simulink model "EPS_sim_test_v8a"  (R2023b)
settings: Solver=FixedStepAuto  StartTime=0.0  StopTime=tsimulation  FixedStep=delta_t  MaxStep=10  RelTol=1e-3
values from neighbouring files (symbols this model uses):
  ADCS =     [RWinfo.mat]
undefined symbols (not defined in the file or in its folder): Bat, Batt, EN, EPS, FIPEX, GPS, OBC, OCS, PL, UHF
libraries: simulink x4, cstextras x2
settings Model: Creator=Ricardo  LastModifiedBy=lricc
settings OptimizationCC: ReuseModelBlockBuffer=off
settings DebuggingCC: AlgebraicLoopMsg=none  UnconnectedInputMsg=warning  UnconnectedOutputMsg=warning  UnconnectedLineMsg=warning
settings ModelReferenceCC: EnableRefExpFcnMdlSchedulingChecks=on
settings SFSimCC: CustomCodeUndefinedFunction=UseInterfaceOnly
settings RTWCC: DLArmComputeVersion=19.05

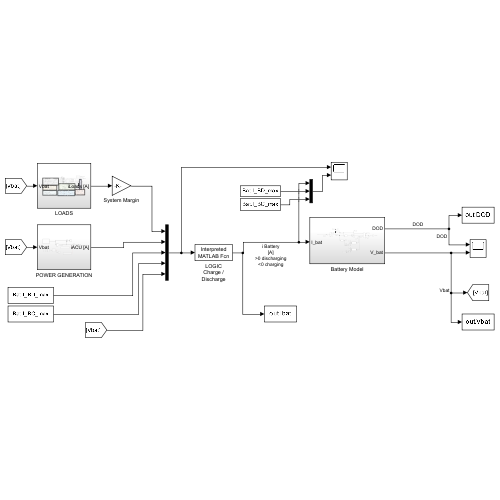
[thumbnail: Simulink's stored preview of the top-level diagram]
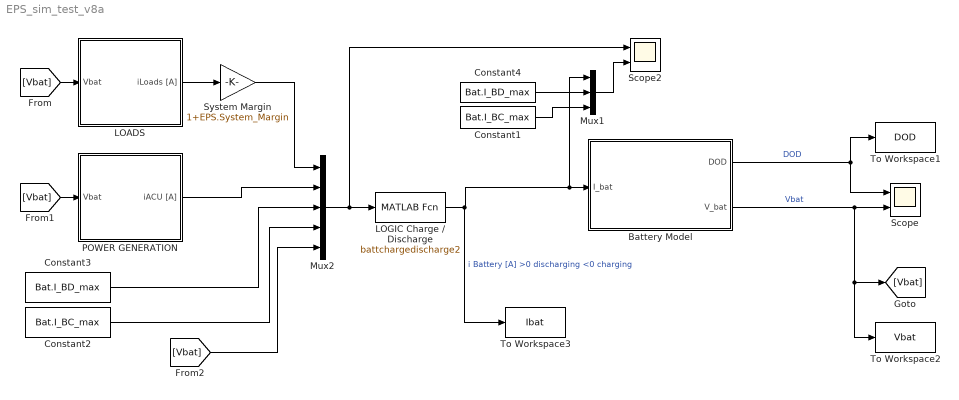
== system EPS_sim_test_v8a ==
  Battery Model : Subsystem
  Constant1 : Constant  Value=Bat.I_BC_max
  Constant2 : Constant  Value=Bat.I_BC_max
  Constant3 : Constant  Value=Bat.I_BD_max
  Constant4 : Constant  Value=Bat.I_BD_max
  LOADS : Subsystem
  LOGIC Charge / Discharge : MATLABFcn  MATLABFcn=battchargedischarge2
  Mux1 : Mux  Inputs=3
  Mux2 : Mux  Inputs=5
  POWER GENERATION : Subsystem
  Scope : Scope  NumInputPorts=2
  Scope2 : Scope  NumInputPorts=2
  System Margin : Gain  Gain=1+EPS.System_Margin
  To Workspace1 : ToWorkspace  VariableName=DOD  SaveFormat=Timeseries  SampleTime=-1
  To Workspace2 : ToWorkspace  VariableName=Vbat  SaveFormat=Timeseries  SampleTime=-1
  To Workspace3 : ToWorkspace  VariableName=Ibat  SaveFormat=Timeseries  SampleTime=-1
  wires:
  Battery Model/2(V_bat) -> [Vbat], To Workspace2/1, Scope/2  "Vbat"
  Battery Model/1(DOD) -> To Workspace1/1, Scope/1  "DOD"
  [Vbat] -> LOADS/1(Vbat)
  POWER GENERATION/1(iACU [A]) -> Mux2/2
  [Vbat] -> POWER GENERATION/1(Vbat)
  LOADS/1(iLoads [A]) -> System Margin/1
  Mux2/1 -> LOGIC Charge / Discharge/1, Scope2/1
  Constant3/1 -> Mux2/3
  Constant2/1 -> Mux2/4
  LOGIC Charge / Discharge/1 -> To Workspace3/1, Battery Model/1(I_bat), Mux1/1  "i Battery [A] >0 discharging <0 charging"
  [Vbat] -> Mux2/5
  Mux1/1 -> Scope2/2
  Constant4/1 -> Mux1/2
  Constant1/1 -> Mux1/3
  System Margin/1 -> Mux2/1

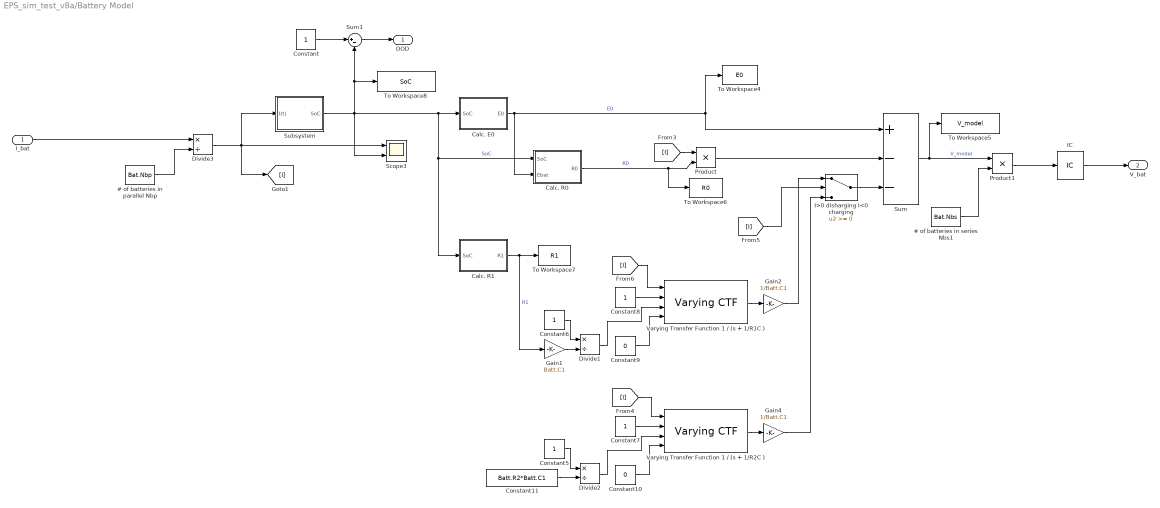
== system EPS_sim_test_v8a/Battery Model ==
  I_bat : Inport
  # of batteries in parallel Nbp : Constant  Value=Bat.Nbp
  # of batteries in series Nbs1 : Constant  Value=Bat.Nbs
  Calc. E0 : MATLAB Function  TreatAsAtomicUnit=on
  Calc. R0 : MATLAB Function  TreatAsAtomicUnit=on
  Calc. R1 : MATLAB Function  TreatAsAtomicUnit=on
  Constant{,5..8} (5 alike) : Constant
  Constant10 : Constant  Value=0
  Constant11 : Constant  Value=Batt.R2*Batt.C1
  Constant9 : Constant  Value=0
  Divide1 : Product  Inputs=*/
  Divide2 : Product  Inputs=*/
  Divide3 : Product  Inputs=*/
  Gain1 : Gain  Gain=Batt.C1
  Gain2 : Gain  Gain=1/Batt.C1
  Gain4 : Gain  Gain=1/Batt.C1
  I>0 disharging I<0 charging : Switch  SaturateOnIntegerOverflow=off  InputSameDT=off
  IC : InitialCondition  Value=4
  Product : Product
  Product1 : Product
  Scope3 : Scope  NumInputPorts=2
  Subsystem : Subsystem
  Sum : Sum  Inputs=+--
  Sum1 : Sum  Inputs=|+-
  To Workspace4 : ToWorkspace  VariableName=E0  SaveFormat=Timeseries  SampleTime=-1
  To Workspace5 : ToWorkspace  VariableName=V_model  SaveFormat=Timeseries  SampleTime=-1
  To Workspace6 : ToWorkspace  VariableName=R0  SaveFormat=Timeseries  SampleTime=-1
  To Workspace7 : ToWorkspace  VariableName=R1  SaveFormat=Timeseries  SampleTime=-1
  To Workspace8 : ToWorkspace  VariableName=SoC  SaveFormat=Timeseries  SampleTime=-1
  Varying Transfer Function 1 / (s + 1/R1C ) : cstextras/Varying CTF  N=1
  Varying Transfer Function 1 / (s + 1/R2C ) : cstextras/Varying CTF  N=1
  DOD : Outport
  V_bat : Outport  Port=2
  wires:
  Varying Transfer Function 1 / (s + 1/R2C )/1 -> Gain4/1
  Constant11/1 -> Divide2/2
  [I] -> Product/1
  Calc. E0/1(E0) -> To Workspace4/1, Sum/1, Calc. R0/2(Ebat)  "E0"
  # of batteries in parallel Nbp/1 -> Divide3/2
  [I] -> I>0 disharging I<0 charging/2
  Divide3/1 -> [I], Subsystem/1(I(t)), Scope3/1
  Calc. R1/1(R1) -> To Workspace7/1, Gain1/1  "R1"
  Calc. R0/1(R0) -> To Workspace6/1, Product/2  "R0"
  Subsystem/1(SoC) -> Sum1/2, To Workspace8/1, Calc. R1/1(SoC), Calc. R0/1(SoC), Calc. E0/1(SoC), Scope3/2  "SoC"
  Product/1 -> Sum/2
  [I] -> Varying Transfer Function 1 / (s + 1/R2C )/1
  Gain4/1 -> I>0 disharging I<0 charging/3
  Sum/1 -> To Workspace5/1, Product1/1  "V_model"
  Constant10/1 -> Varying Transfer Function 1 / (s + 1/R2C )/4
  Gain2/1 -> I>0 disharging I<0 charging/1
  Constant5/1 -> Divide2/1
  Constant8/1 -> Varying Transfer Function 1 / (s + 1/R1C )/2
  Varying Transfer Function 1 / (s + 1/R1C )/1 -> Gain2/1
  [I] -> Varying Transfer Function 1 / (s + 1/R1C )/1
  Constant6/1 -> Divide1/1
  Constant7/1 -> Varying Transfer Function 1 / (s + 1/R2C )/2
  Divide1/1 -> Varying Transfer Function 1 / (s + 1/R1C )/3
  Constant9/1 -> Varying Transfer Function 1 / (s + 1/R1C )/4
  I>0 disharging I<0 charging/1 -> Sum/3
  Product1/1 -> IC/1
  Gain1/1 -> Divide1/2
  Divide2/1 -> Varying Transfer Function 1 / (s + 1/R2C )/3
  # of batteries in series Nbs1/1 -> Product1/2
  I_bat/1 -> Divide3/1
  Constant/1 -> Sum1/1
  Sum1/1 -> DOD/1
  IC/1 -> V_bat/1

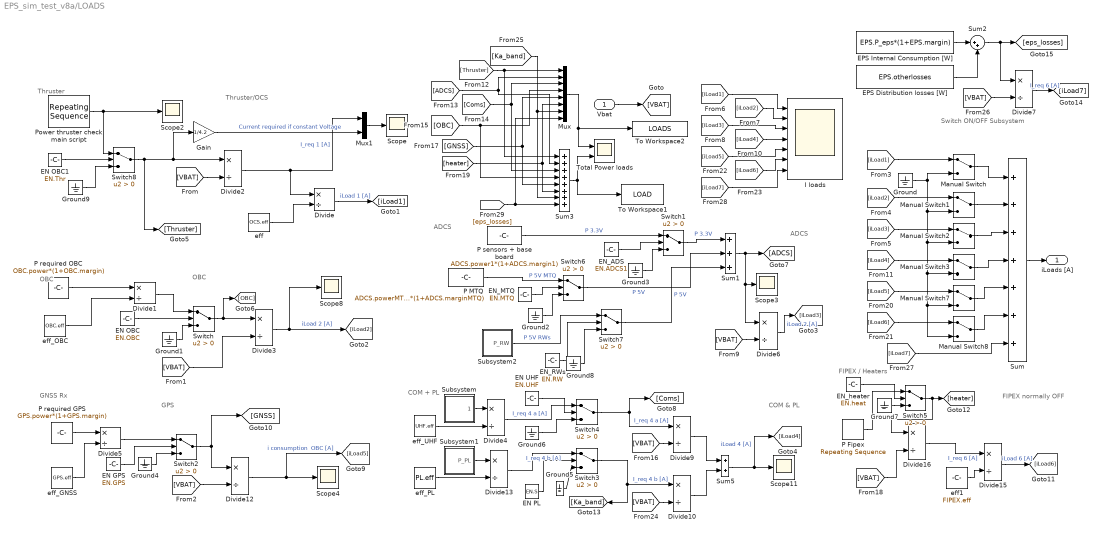
== system EPS_sim_test_v8a/LOADS ==
  note: Switch
      | ON/OFF
      | Subsystem
  note: FIPEX / Heaters
  note: COM + PL
  note: ADCS
  note: OBC
  note: Thruster
  note: Thruster/OCS
  note: OBC
  note: ADCS
  note: COM & PL
  note: GPS
  note: GNSS Rx
  note: FIPEX
      | normally
      | OFF
  Vbat : Inport
  Divide{,1..7,9..10,12..13,15..16} (14 alike) : Product  Inputs=*/
  EN GPS : Constant  Value=EN.GPS
  EN OBC : Constant  Value=EN.OBC
  EN OBC1 : Constant  Value=EN.Thr
  EN PL : Constant  Value=EN.S
  EN UHF : Constant  Value=EN.UHF
  EN_ADS : Constant  Value=EN.ADCS1
  EN_MTQ : Constant  Value=EN.MTQ
  EN_RWs : Constant  Value=EN.RW
  EN_heater : Constant  Value=EN.heat
  EPS Distribution losses [W] : Constant  Value=EPS.otherlosses
  EPS Internal Consumption [W] : Constant  Value=EPS.P_eps*(1+EPS.margin)
  Gain : Gain  Gain=1/4.2
  Ground{,1..9} (10 alike) : Ground
  I loads : Scope  NumInputPorts=7
  Manual Switch{,1..3,7..8} (6 alike) : ManualSwitch
  Mux : Mux  Inputs=8
  Mux1 : Mux  Inputs=2
  P Fipex : simulink/Sources/Repeating Sequence  rep_seq_t=FIPEX.t_Fi  rep_seq_y=FIPEX.p_Fi*(1+FIPEX.margin)
  P MTQ : Constant  Value=ADCS.powerMTQ/ADCS.effMTQ *(1+ADCS.marginMTQ)
  P required GPS : Constant  Value=GPS.power*(1+GPS.margin)
  P required OBC : Constant  Value=OBC.power*(1+OBC.margin)
  P sensors + base board : Constant  Value=ADCS.power1*(1+ADCS.margin1)
  Power thruster check main script : simulink/Sources/Repeating Sequence  rep_seq_t=OCS.t_thr  rep_seq_y=OCS.p_thr*(1+OCS.margin)
  Scope{,2..4,8,11} (6 alike) : Scope
  Subsystem : Subsystem
  Subsystem1 : Subsystem
  Subsystem2 : Subsystem
  Sum : Sum  Inputs=+++++++
  Sum1 : Sum  Inputs=+++
  Sum2 : Sum  Inputs=|++
  Sum3 : Sum  Inputs=++++++++
  Sum5 : Sum
  Switch{,1..8} (9 alike) : Switch  Criteria=u2 > Threshold  SaturateOnIntegerOverflow=off  InputSameDT=off
  To Workspace1 : ToWorkspace  VariableName=LOAD  SaveFormat=Timeseries  SampleTime=-1
  To Workspace2 : ToWorkspace  VariableName=LOADS  SaveFormat=Timeseries  SampleTime=-1
  Total Power loads : Scope  NumInputPorts=2
  eff : Constant  Value=OCS.eff
  eff1 : Constant  Value=FIPEX.eff
  eff_GNSS : Constant  Value=GPS.eff
  eff_OBC : Constant  Value=OBC.eff
  eff_PL : Constant  Value=PL.eff
  eff_UHF : Constant  Value=UHF.eff
  iLoads [A] : Outport
  wires:
  Gain/1 -> Mux1/2  "Current required if constant Voltage"
  Divide2/1 -> Divide/1, Mux1/1  "I_req 1 [A]"
  [VBAT] -> Divide3/2
  Vbat/1 -> [VBAT]
  [VBAT] -> Divide2/2
  Sum/1 -> iLoads [A]/1
  Mux1/1 -> Scope/1
  eff_OBC/1 -> Divide1/2
  Switch8/1 -> [Thruster], Gain/1, Divide2/1
  eff/1 -> Divide/2
  Divide/1 -> [iLoad1]  "iLoad 1 [A]"
  Manual Switch/1 -> Sum/1
  Manual Switch1/1 -> Sum/2
  Manual Switch2/1 -> Sum/3
  [iLoad2] -> I loads/2
  [iLoad1] -> I loads/1
  [iLoad3] -> I loads/3
  [iLoad4] -> I loads/4
  Manual Switch3/1 -> Sum/4
  Subsystem/1(P_UHF) -> Divide4/1
  [iLoad4] -> Manual Switch3/1
  [iLoad3] -> Manual Switch2/1
  [iLoad2] -> Manual Switch1/1
  [iLoad1] -> Manual Switch/1
  Ground/1 -> Manual Switch/2, Manual Switch8/2, Manual Switch7/2, Manual Switch3/2, Manual Switch2/2, Manual Switch1/2
  Mux/1 -> To Workspace2/1, Total Power loads/1
  [Thruster] -> Sum3/1, Mux/1
  [ADCS] -> Mux/2, Sum3/2
  [Coms] -> Sum3/3, Mux/3
  [OBC] -> Sum3/4, Mux/4
  [heater] -> Sum3/6, Mux/6
  Sum3/1 -> To Workspace1/1, Total Power loads/2
  Divide12/1 -> [iLoad5], Scope4/1  "i consumption  OBC [A]"
  [VBAT] -> Divide12/2
  eff_GNSS/1 -> Divide5/2
  [GNSS] -> Sum3/5, Mux/5
  eff1/1 -> Divide15/2
  Divide15/1 -> [iLoad6]  "iLoad 6 [A]"
  P Fipex/1 -> Switch5/1
  Divide16/1 -> Divide15/1  "I_req 6 [A]"
  [VBAT] -> Divide16/2
  Switch5/1 -> Divide16/1, [heater]
  Manual Switch7/1 -> Sum/5
  Manual Switch8/1 -> Sum/6
  [iLoad6] -> Manual Switch8/1
  [iLoad5] -> Manual Switch7/1
  [iLoad5] -> I loads/5
  [iLoad6] -> I loads/6
  Switch1/1 -> Sum1/1  "P 3.3V"
  P required OBC/1 -> Divide1/1
  Switch/1 -> [OBC], Divide3/1
  Divide3/1 -> Scope8/1, [iLoad2]  "iLoad 2 [A]"
  P required GPS/1 -> Divide5/1
  Switch2/1 -> [GNSS], Divide12/1
  Subsystem1/1(P_PL) -> Divide13/1
  eff_PL/1 -> Divide13/2
  Switch4/1 -> [Coms], Divide9/1  "I_req 4 a [A]"
  Switch3/1 -> Divide10/1, [Ka_band]  "I_req 4 b [A]"
  eff_UHF/1 -> Divide4/2
  [VBAT] -> Divide9/2
  [VBAT] -> Divide10/2
  Divide10/1 -> Sum5/2
  Divide9/1 -> Sum5/1
  [VBAT] -> Divide6/2
  Divide6/1 -> [iLoad3]  "iLoad 2 [A]"
  Divide1/1 -> Switch/1
  EN OBC/1 -> Switch/2
  Ground1/1 -> Switch/3
  Ground4/1 -> Switch2/3
  EN GPS/1 -> Switch2/2
  Divide5/1 -> Switch2/1
  Ground5/1 -> Switch3/3
  EN PL/1 -> Switch3/2
  EN UHF/1 -> Switch4/2
  Ground6/1 -> Switch4/3
  Divide4/1 -> Switch4/1  "I_req 4 a [A]"
  Divide13/1 -> Switch3/1  "I_req 4 b [A]"
  Ground7/1 -> Switch5/3
  EN_heater/1 -> Switch5/2
  Ground3/1 -> Switch1/3
  EN_ADS/1 -> Switch1/2
  P sensors + base board/1 -> Switch1/1  "P 3.3V"
  Ground9/1 -> Switch8/3
  EN OBC1/1 -> Switch8/2
  Power thruster check main script/1 -> Scope2/1, Switch8/1
  Sum5/1 -> [iLoad4], Scope11/1  "iLoad 4 [A]"
  [Ka_band] -> Sum3/7, Mux/7
  EN_MTQ/1 -> Switch6/2
  Ground2/1 -> Switch6/3
  Ground8/1 -> Switch7/3
  EN_RWs/1 -> Switch7/2
  Subsystem2/1(P_RW) -> Switch7/1  "P 5V RWs"
  Sum1/1 -> Divide6/1, Scope3/1, [ADCS]
  Switch6/1 -> Sum1/2  "P 5V"
  Switch7/1 -> Sum1/3  "P 5V"
  P MTQ/1 -> Switch6/1  "P 5V MTQ"
  EPS Internal Consumption [W]/1 -> Sum2/1
  EPS Distribution losses [W]/1 -> Sum2/2
  [VBAT] -> Divide7/2
  Sum2/1 -> [eps_losses], Divide7/1
  Divide7/1 -> [iLoad7]  "I_req 6 [A]"
  [iLoad7] -> Sum/7
  [iLoad7] -> I loads/7
  [eps_losses] -> Mux/8, Sum3/8

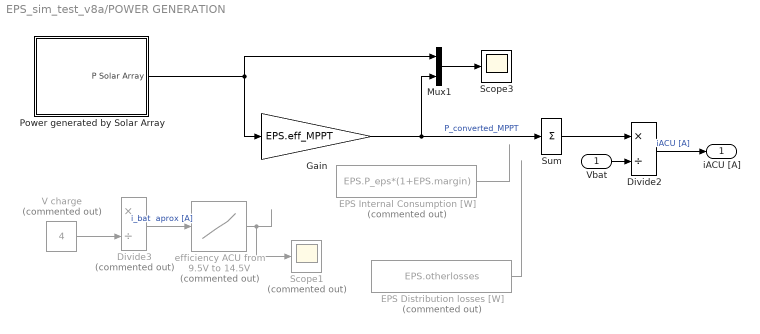
== system EPS_sim_test_v8a/POWER GENERATION ==
  Vbat : Inport
  Divide2 : Product  Inputs=*/
  Divide3 : Product  Commented=on  Inputs=*/
  EPS Distribution losses [W] : Constant  Commented=on  Value=EPS.otherlosses
  EPS Internal Consumption [W] : Constant  Commented=on  Value=EPS.P_eps*(1+EPS.margin)
  Gain : Gain  Gain=EPS.eff_MPPT
  Mux1 : Mux  Inputs=2
  Power generated by Solar Array : Subsystem
  Scope1 : Scope  Commented=on
  Scope3 : Scope
  Sum : Sum  Inputs=+
  V charge : Constant  Commented=on  Value=4
  efficiency ACU from 9.5V to 14.5V : Lookup_n-D  Commented=on  NumberOfTableDimensions=1  BreakpointsForDimension1=[0,0.13,0.16,0.236,0.4187,0.654,0.684,0.745,0.801,0.9372,1.046,1.16,1.21,1.5,1.66,2,4]  Table=[0.905,0.928,0.9296,0.9296,0.9337,0.9296,0.9296,0.9296,0.9275,0.9275,0.9254,0.9254,0.9234,0.9193,0.9193,0.9134,0.9134]  InternalRulePriority=Speed  RndMeth=Simplest
  iACU [A] : Outport
  wires:
  Divide2/1 -> iACU [A]/1  "iACU [A]"
  Mux1/1 -> Scope3/1
  Vbat/1 -> Divide2/2
  efficiency ACU from 9.5V to 14.5V/1 -> Scope1/1
  Gain/1 -> Mux1/2, Sum/1  "P_converted_MPPT"
  Sum/1 -> Divide2/1
  EPS Internal Consumption [W]/1 -> ?
  Divide3/1 -> efficiency ACU from 9.5V to 14.5V/1  "i_bat  aprox [A]"
  V charge/1 -> Divide3/2
  Power generated by Solar Array/1(P Solar Array) -> Gain/1, Mux1/1
  EPS Distribution losses [W]/1 -> ?

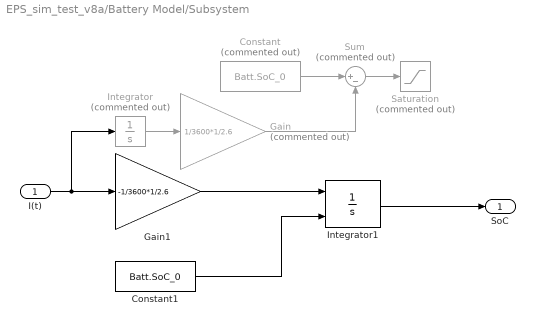
== system EPS_sim_test_v8a/Battery Model/Subsystem ==
  I(t) : Inport
  Constant : Constant  Commented=on  Value=Batt.SoC_0
  Constant1 : Constant  Value=Batt.SoC_0
  Gain : Gain  Commented=on  Gain=1/3600*1/2.6
  Gain1 : Gain  Gain=-1/3600*1/2.6
  Integrator : Integrator  Commented=on
  Integrator1 : Integrator  InitialConditionSource=external  LimitOutput=on  UpperSaturationLimit=1  LowerSaturationLimit=0
  Saturation : Saturate  Commented=on  UpperLimit=1  LowerLimit=0
  Sum : Sum  Commented=on  Inputs=|+-
  SoC : Outport
  wires:
  I(t)/1 -> Integrator/1, Gain1/1
  Integrator/1 -> Gain/1
  Gain/1 -> Sum/2
  Sum/1 -> Saturation/1
  Constant/1 -> Sum/1
  Integrator1/1 -> SoC/1
  Constant1/1 -> Integrator1/2
  Gain1/1 -> Integrator1/1

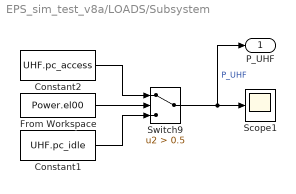
== system EPS_sim_test_v8a/LOADS/Subsystem ==
  Constant1 : Constant  Value=UHF.pc_idle
  Constant2 : Constant  Value=UHF.pc_access
  From Workspace : FromWorkspace  VariableName=Power.el00
  Scope1 : Scope
  Switch9 : Switch  Criteria=u2 > Threshold  Threshold=0.5  SaturateOnIntegerOverflow=off  InputSameDT=off
  P_UHF : Outport
  wires:
  Constant2/1 -> Switch9/1
  From Workspace/1 -> Switch9/2
  Constant1/1 -> Switch9/3
  Switch9/1 -> P_UHF/1, Scope1/1  "P_UHF"

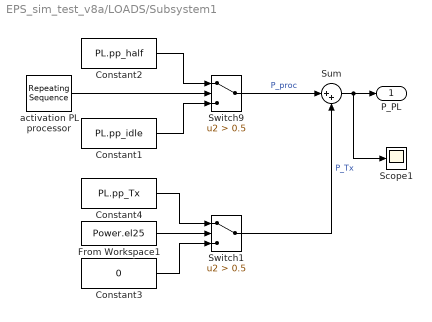
== system EPS_sim_test_v8a/LOADS/Subsystem1 ==
  Constant1 : Constant  Value=PL.pp_idle
  Constant2 : Constant  Value=PL.pp_half
  Constant3 : Constant  Value=0
  Constant4 : Constant  Value=PL.pp_Tx
  From Workspace1 : FromWorkspace  VariableName=Power.el25
  Scope1 : Scope
  Sum : Sum  Inputs=|++
  Switch1 : Switch  Criteria=u2 > Threshold  Threshold=0.5  SaturateOnIntegerOverflow=off  InputSameDT=off
  Switch9 : Switch  Criteria=u2 > Threshold  Threshold=0.5  SaturateOnIntegerOverflow=off  InputSameDT=off
  activation PL processor : simulink/Sources/Repeating Sequence  rep_seq_t=Power.tout  rep_seq_y=PL.active
  P_PL : Outport
  wires:
  Constant2/1 -> Switch9/1
  activation PL processor/1 -> Switch9/2
  Constant1/1 -> Switch9/3
  Switch9/1 -> Sum/1  "P_proc"
  Sum/1 -> Scope1/1, P_PL/1
  Constant4/1 -> Switch1/1
  Constant3/1 -> Switch1/3
  From Workspace1/1 -> Switch1/2
  Switch1/1 -> Sum/2  "P_Tx"

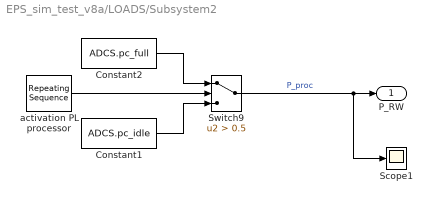
== system EPS_sim_test_v8a/LOADS/Subsystem2 ==
  Constant1 : Constant  Value=ADCS.pc_idle
  Constant2 : Constant  Value=ADCS.pc_full
  Scope1 : Scope
  Switch9 : Switch  Criteria=u2 > Threshold  Threshold=0.5  SaturateOnIntegerOverflow=off  InputSameDT=off
  activation PL processor : simulink/Sources/Repeating Sequence  rep_seq_t=Power.tout  rep_seq_y=ADCS.RWactive
  P_RW : Outport
  wires:
  Constant2/1 -> Switch9/1
  activation PL processor/1 -> Switch9/2
  Constant1/1 -> Switch9/3
  Switch9/1 -> Scope1/1, P_RW/1  "P_proc"

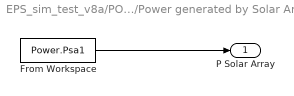
== system EPS_sim_test_v8a/POWER GENERATION/Power generated by Solar Array ==
  From Workspace : FromWorkspace  VariableName=Power.Psa1
  P Solar Array : Outport
  wires:
  From Workspace/1 -> P Solar Array/1

== matlab function EPS_sim_test_v8a/Battery Model/Calc. E0 ==
  data: SoC input; E0 output
function E0 = fcn(SoC)
ebat0 = 3.288;
ebat1 = 1.813;
ebat2 = -4.205;
ebat3 = 5.306;
ebat4 = -2.03;

E0 = ebat0 + ebat1.*SoC + ebat2.*SoC^2 + ebat3.*SoC^3 + ebat4.*SoC^4;

== matlab function EPS_sim_test_v8a/Battery Model/Calc. R1 ==
  data: SoC input; R1 output
function R1 = fcn(SoC)
dint0 = 0.065;
dint1 = -0.057;
dint2 = -0.029;
dint3 = 0.161;
dint4 = -0.116;

R1 = dint0 + dint1.*SoC + dint2.*SoC^2 + dint3.*SoC^3 + dint4.*SoC^4;

== matlab function EPS_sim_test_v8a/Battery Model/Calc. R0 ==
  data: SoC input; R0 output; Ebat input
function R0 = fcn(SoC,Ebat)
rsint0 = 0.053;
rsint1 = 0.005;
rsint2 = 0.004;
rsint3 = -2;
rsint4 = 3.6;

R0 = rsint0 + rsint1*Ebat + rsint2*exp(rsint3*(Ebat-rsint4));
